simulink model "task1simlink1"  (R2018a)
settings: Solver=VariableStepAuto  StartTime=0.0  StopTime=10.0  RelTol=1e-3
settings Model: Creator=SRKR EEE  LastModifiedBy=SRKR EEE

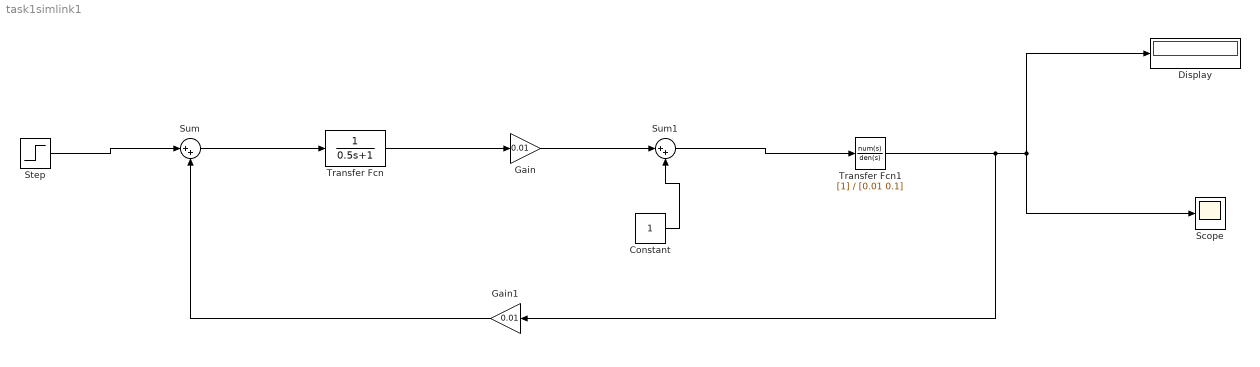
== system task1simlink1 ==
  Constant : Constant
  Display : Display
  Gain : Gain  Gain=0.01
  Gain1 : Gain  Gain=0.01
  Scope : Scope
  Step : Step  SampleTime=0
  Sum : Sum  Inputs=|++
  Sum1 : Sum  Inputs=|++
  Transfer Fcn : TransferFcn  Denominator=[0.5 1]
  Transfer Fcn1 : TransferFcn  Denominator=[0.01 0.1]
  wires:
  Step/1 -> Sum/1
  Sum/1 -> Transfer Fcn/1
  Transfer Fcn/1 -> Gain/1
  Gain/1 -> Sum1/1
  Sum1/1 -> Transfer Fcn1/1
  Transfer Fcn1/1 -> Gain1/1, Scope/1, Display/1
  Gain1/1 -> Sum/2
  Constant/1 -> Sum1/2
